simulink subsystem "HbridgeSub"  (R2023b)
settings: Solver=VariableStepAuto  StartTime=0.0  StopTime=10.0  RelTol=1e-3
libraries: spsMosfetLib x4
settings Model: Creator=mukoo  LastModifiedBy=mukoo

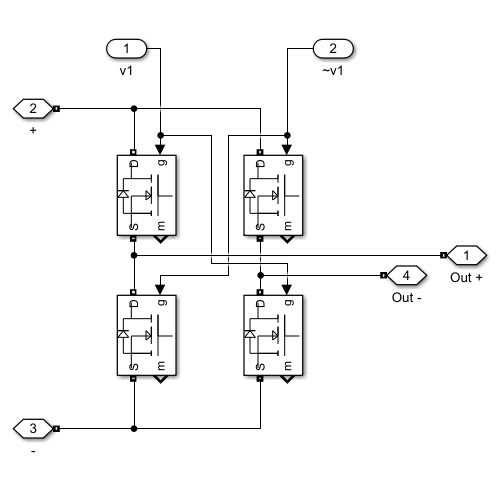
[thumbnail: Simulink's stored preview of the top-level diagram]
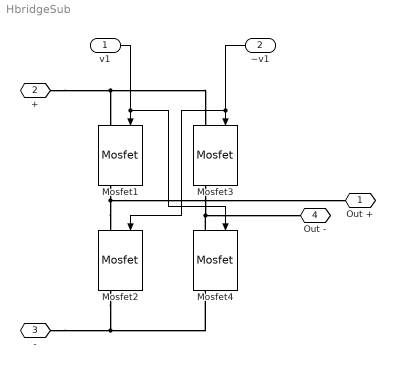
== system HbridgeSub ==
  v1 : Inport
  ~v1 : Inport  Port=2
  Mosfet{1..4} (4 alike) : spsMosfetLib/Mosfet  Ron=0.1  Lon=0  Rd=0.01  Vfd=0  IC=0  Rs=1e5  Cs=inf  Measurements=on
  Out + : PMIOPort  Side=Right
  + : PMIOPort  Port=2  Side=Left
  - : PMIOPort  Port=3  Side=Left
  Out - : PMIOPort  Port=4  Side=Right
  wires:
  v1/1 -> Mosfet4/1, Mosfet1/1
  ~v1/1 -> Mosfet2/1, Mosfet3/1
  connections:
  Mosfet4/RConn1 -- Mosfet2/RConn1 -- -/RConn1
  Mosfet3/RConn1 -- Mosfet4/LConn1 -- Out -/RConn1
  Mosfet2/LConn1 -- Mosfet1/RConn1 -- Out +/RConn1
  Mosfet3/LConn1 -- Mosfet1/LConn1 -- +/RConn1
